simulink model "LTI_test"  (R2020b)
settings: Solver=VariableStepAuto  StartTime=0.0  StopTime=Tsim  RelTol=1e-3
values from neighbouring files (symbols this model uses):
  a = B(2,1)    [getMatrices.m]
  A = [0, 1, 0, 0 ... (first row only)    [ErrorStateMatrices.m]    (also in getMatrices.m = [)
  B = [Bswa Bcurv]    [ErrorStateMatrices.m]    (also in getMatrices.m = [0, 2*Cf/m, 0, 2*Cf*lf/Jz; 0, 0 , 0, 2*d*Csf/Jz]')
  Cf = VEHICLE.CORNERING_STIFF    [ErrorStateMatrices.m]    (also in LoadVehicleParameters.m = 72705; RunSimulation.m; getMatrices.m = 72705)
  collecting_data = controller_input(end)    [LTI_MPC.m]    (also in RunSimulation.m = 0)
  Cr = Cf    [ErrorStateMatrices.m]    (also in LoadVehicleParameters.m = 72705; RunSimulation.m; getMatrices.m = 72705)
  DLCoffset = round(vx*3.6/60*250,-1)    [RunSimulation.m]
  Iz = VEHICLE.INERTIA_Z    [RunSimulation.m]
  L = controller_input(end-2)    [LTI_MPC.m]    (also in RunSimulation.m = 15)
  lambda_alpha = 0.2    [RunSimulation.m]
  lambda_slack = 1e6    (= 1000000)    [RunSimulation.m]
  lf = VEHICLE.LF    [ErrorStateMatrices.m]    (also in LoadVehicleParameters.m = 1.311; RunSimulation.m; getMatrices.m = 1.311)
  lr = VEHICLE.LR    [ErrorStateMatrices.m]    (also in LoadVehicleParameters.m = 1.311; RunSimulation.m; getMatrices.m = 1.311)
  m = VEHICLE.MASS    [ErrorStateMatrices.m]    (also in LoadVehicleParameters.m = 1599.98; RunSimulation.m; getMatrices.m = 1599.98)
  N = T_test/Ts    (= 100)    [RunSimulation.m]    (also in nominalMPC.m = u(end))
  n = controller_input(end-1)    [LTI_MPC.m]    (also in RunSimulation.m = 4)
  nu = 2    [LTI_MPC.m]    (also in RunSimulation.m; nominalMPC.m = 1)
  ny = 2    [LTI_MPC.m]    (also in RunSimulation.m)
  Ts = 0.05    [RunSimulation.m]    (also in getMatrices.m = 0.1)
  vx = controller_input(2)    [LTI_MPC.m]    (also in RunSimulation.m = 22.2222222222)
undefined symbols (not defined in the file or in its folder): DDPC, DiscIntNeverNeededParam, nominalMPC, VEHICLE
libraries: simulink x2
settings Model: Creator=LAMES Workstation  LastModifiedBy=LAMES Workstation

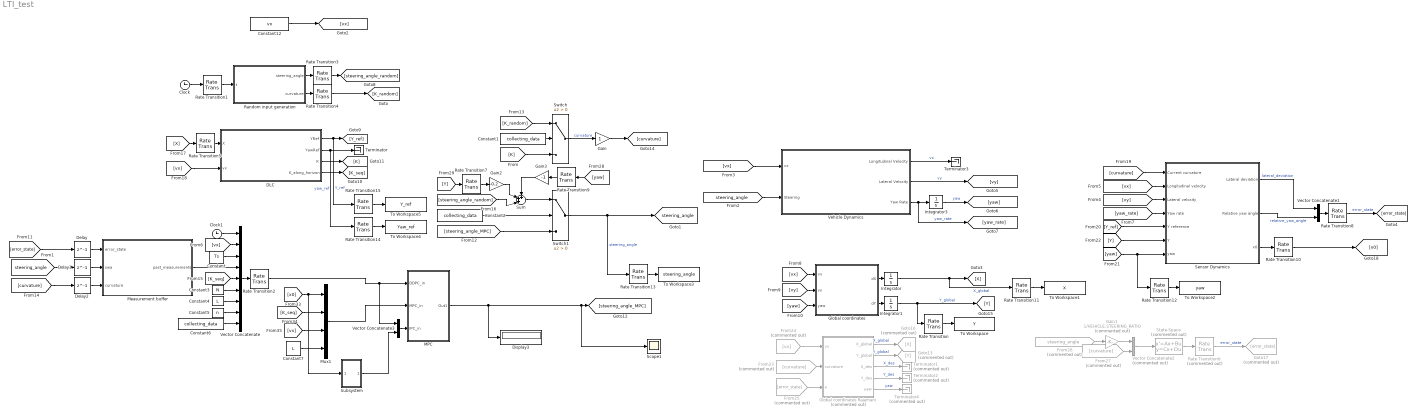
== system LTI_test ==
  Clock : Clock
  Clock1 : Clock
  Constant : Constant  Value=Ts  SampleTime=Ts
  Constant1 : Constant  Value=collecting_data  SampleTime=Ts
  Constant12 : Constant  Value=vx  SampleTime=Ts
  Constant2 : Constant  Value=collecting_data  SampleTime=Ts
  Constant3 : Constant  Value=N  SampleTime=Ts
  Constant4 : Constant  Value=L  SampleTime=Ts
  Constant5 : Constant  Value=n  SampleTime=Ts
  Constant6 : Constant  Value=collecting_data  SampleTime=Ts
  Constant7 : Constant  Value=L  SampleTime=Ts
  DLC : MATLAB Function  TreatAsAtomicUnit=on
  Delay : Delay  DelayLength=1  InitialCondition=0  SampleTime=Ts
  Delay1 : Delay  DelayLength=1  InitialCondition=0  SampleTime=Ts
  Delay2 : Delay  DelayLength=1  InitialCondition=0  SampleTime=Ts
  Display3 : Display
  From23 : From  Commented=on  GotoTag=curvature
  From24 : From  Commented=on  GotoTag=vx
  From25 : From  Commented=on  GotoTag=error_state
  From26 : From  Commented=on  GotoTag=steering_angle  TagVisibility=global
  From27 : From  Commented=on  GotoTag=curvature
  Gain : Gain
  Gain1 : Gain  Commented=on  Gain=1/VEHICLE.STEERING_RATIO
  Gain2 : Gain  Gain=-0.2
  Gain3 : Gain  Gain=-1
  Global coordinates : MATLAB Function  TreatAsAtomicUnit=on
  Global coordinates Rajamani : Subsystem  Commented=on
  Goto13 : Goto  Commented=on  GotoTag=Y
  Goto16 : Goto  Commented=on  GotoTag=X
  Goto17 : Goto  Commented=on  GotoTag=error_state
  Integrator : Integrator
  Integrator1 : Integrator
  Integrator3 : Integrator
  MPC : Subsystem  Variant=on
  Measurement buffer : MATLAB Function  TreatAsAtomicUnit=on
  Mux1 : Mux
  Random input generation : MATLAB Function  TreatAsAtomicUnit=on
  Rate Transition{,11..15} (6 alike) : RateTransition  InitialCondition=Ts
  Rate Transition1 : RateTransition  OutPortSampleTime="5*Ts  % hold the input for a few samples"
  Rate Transition{2..5,7..10} (8 alike) : RateTransition  OutPortSampleTime=Ts
  Rate Transition6 : RateTransition  Commented=on  OutPortSampleTime=Ts
  Scope1 : Scope
  Sensor Dynamics : Subsystem
  State-Space : StateSpace  Commented=on  A=A  B=B  C=[1 0 0 0; 0 0 1 0]  D=zeros(2)  InitialCondition=0
  Subsystem : Subsystem
  Sum : Sum  Inputs=+++|
  Switch : Switch  Criteria=u2 > Threshold
  Switch1 : Switch  Criteria=u2 > Threshold
  Terminator : Terminator
  Terminator1 : Terminator  Commented=on
  Terminator2 : Terminator  Commented=on
  Terminator3 : Terminator
  Terminator4 : Terminator  Commented=on
  To Workspace : ToWorkspace  VariableName=Y  SaveFormat=Timeseries  SampleTime=-1
  To Workspace1 : ToWorkspace  VariableName=X  SaveFormat=Timeseries  SampleTime=-1
  To Workspace2 : ToWorkspace  VariableName=yaw  SaveFormat=Timeseries  SampleTime=-1
  To Workspace3 : ToWorkspace  VariableName=steering_angle  SaveFormat=Timeseries  SampleTime=-1
  To Workspace4 : ToWorkspace  VariableName=Yaw_ref  SaveFormat=Timeseries  SampleTime=-1
  To Workspace5 : ToWorkspace  VariableName=Y_ref  SaveFormat=Timeseries  SampleTime=-1
  Vector Concatenate : Concatenate  NumInputs=9
  Vector Concatenate1 : Concatenate
  Vector Concatenate2 : Concatenate  Commented=on
  Vector Concatenate3 : Concatenate
  Vehicle Dynamics : Subsystem
  tag scope: steering_angle=global
  wires:
  Constant4/1 -> Vector Concatenate/7
  Constant5/1 -> Vector Concatenate/8
  [K_seq] -> Vector Concatenate/5
  Constant6/1 -> Vector Concatenate/9
  Constant3/1 -> Vector Concatenate/6
  Vector Concatenate/1 -> Rate Transition2/1
  [vx] -> Vector Concatenate/2
  Constant/1 -> Vector Concatenate/3
  Clock1/1 -> Vector Concatenate/1
  Measurement buffer/1(past_measurements) -> Vector Concatenate/4
  Constant1/1 -> Switch/2
  Gain/1 -> [curvature]
  [K_random] -> Switch/1
  [K] -> Switch/3
  Switch/1 -> Gain/1  "curvature"
  [steering_angle_MPC] -> Switch1/3
  Constant2/1 -> Switch1/2
  Switch1/1 -> Rate Transition13/1, [steering_angle]  "steering_angle"
  [steering_angle] -> Vehicle Dynamics/2(Steering)
  Vehicle Dynamics/1(Longitudinal Velocity) -> Terminator3/1  "vx"
  [vx] -> Vehicle Dynamics/1(vx)
  Constant12/1 -> [vx]
  [vy] -> Sensor Dynamics/3(Lateral velocity)
  [vx] -> Sensor Dynamics/2(Longitudinal velocity)
  [yaw_rate] -> Sensor Dynamics/4(Yaw rate)
  [yaw] -> Global coordinates/3(yaw)
  Integrator1/1 -> Rate Transition/1, [Y]  "Y_global"
  Global coordinates/2(dY) -> Integrator1/1
  Integrator/1 -> Rate Transition11/1, [X]  "X_global"
  [vx] -> Global coordinates/1(vx)
  [vy] -> Global coordinates/2(vy)
  Global coordinates/1(dX) -> Integrator/1
  Vector Concatenate1/1 -> Rate Transition8/1
  Sensor Dynamics/1(Lateral deviation) -> Vector Concatenate1/1  "lateral_deviation"
  Sensor Dynamics/2(Relative yaw angle) -> Vector Concatenate1/2  "relative_yaw_angle"
  DLC/3(K) -> [K]
  DLC/2(YawRef) -> Rate Transition14/1, Terminator/1  "yaw_ref"
  [vx] -> DLC/2(vx)
  DLC/4(K_along_horizon) -> [K_seq]
  DLC/1(YRef) -> Rate Transition15/1, [Y_ref]  "Y_ref"
  [curvature] -> Sensor Dynamics/1(Current curvature)
  Vehicle Dynamics/2(Lateral Velocity) -> [vy]  "vy"
  Integrator3/1 -> [yaw]  "yaw"
  Vehicle Dynamics/3(Yaw Rate) -> [yaw_rate], Integrator3/1  "yaw_rate"
  Rate Transition8/1 -> [error_state]  "error_state"
  [Y_ref] -> Sensor Dynamics/5(Y reference)
  [Y] -> Sensor Dynamics/6(Y)
  [yaw] -> Rate Transition12/1, Sensor Dynamics/7(yaw)
  [X] -> Rate Transition5/1
  Rate Transition5/1 -> DLC/1(X)
  From23/1 -> Global coordinates Rajamani/2(curvature)
  From24/1 -> Global coordinates Rajamani/1(vx)
  Global coordinates Rajamani/1(X_global) -> Goto16/1  "X_global"
  Global coordinates Rajamani/2(Y_global) -> Goto13/1  "Y_global"
  From25/1 -> Global coordinates Rajamani/3(e)
  Global coordinates Rajamani/3(X_des) -> Terminator1/1  "X_des"
  Global coordinates Rajamani/4(Y_des) -> Terminator2/1  "Y_des"
  From27/1 -> Vector Concatenate2/2
  Vector Concatenate2/1 -> State-Space/1
  State-Space/1 -> Rate Transition6/1
  Rate Transition6/1 -> Goto17/1  "error_state"
  Global coordinates Rajamani/5(yaw) -> Terminator4/1  "yaw"
  From26/1 -> Gain1/1
  Gain1/1 -> Vector Concatenate2/1
  Rate Transition2/1 -> Vector Concatenate3/1, MPC/1(DDPC_in)
  [error_state] -> Delay/1
  Delay/1 -> Measurement buffer/1(error_state)
  [steering_angle] -> Delay1/1
  Delay1/1 -> Measurement buffer/2(swa)
  [curvature] -> Delay2/1
  Delay2/1 -> Measurement buffer/3(curvature)
  [steering_angle_random] -> Sum/3
  Sum/1 -> Switch1/1
  Rate Transition7/1 -> Gain2/1
  Gain2/1 -> Sum/2
  [Y] -> Rate Transition7/1
  [yaw] -> Rate Transition9/1
  Rate Transition9/1 -> Gain3/1
  Gain3/1 -> Sum/1
  Sensor Dynamics/3(x0) -> Rate Transition10/1
  Rate Transition10/1 -> [x0]
  Rate Transition/1 -> To Workspace/1
  Rate Transition11/1 -> To Workspace1/1
  Rate Transition12/1 -> To Workspace2/1
  Rate Transition13/1 -> To Workspace3/1
  Rate Transition14/1 -> To Workspace4/1
  Rate Transition15/1 -> To Workspace5/1
  MPC/1(Out1) -> Display3/1, Scope1/1, [steering_angle_MPC]
  [vx] -> Mux1/3
  Mux1/1 -> MPC/2(MPC_in)
  [K_seq] -> Mux1/2
  [x0] -> Subsystem/1(In1), Mux1/1
  Rate Transition4/1 -> [K_random]
  Random input generation/2(curvature) -> Rate Transition4/1
  Clock/1 -> Rate Transition1/1
  Rate Transition3/1 -> [steering_angle_random]
  Rate Transition1/1 -> Random input generation/1(t)
  Random input generation/1(steering_angle) -> Rate Transition3/1
  Constant7/1 -> Mux1/4
  Vector Concatenate3/1 -> MPC/3(IPC_in)
  Subsystem/1(Out1) -> Vector Concatenate3/2

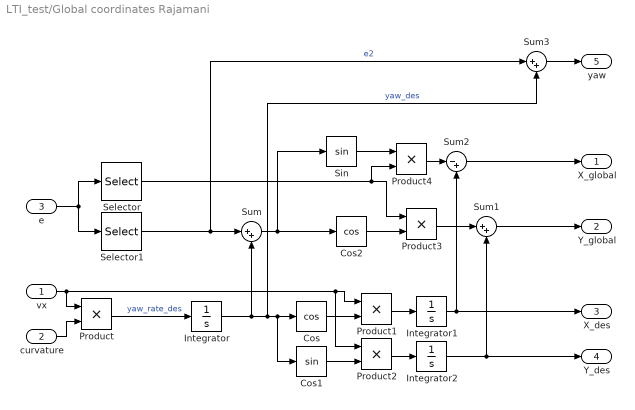
== system LTI_test/Global coordinates Rajamani ==
  vx : Inport
  curvature : Inport  Port=2
  e : Inport  Port=3
  Cos : Trigonometry  Operator=cos
  Cos1 : Trigonometry
  Cos2 : Trigonometry  Operator=cos
  Integrator : Integrator
  Integrator1 : Integrator
  Integrator2 : Integrator
  Product{,1..4} (5 alike) : Product
  Selector : Selector  InputPortWidth=2  IndexOptions=Index vector (dialog)  Indices=1  OutputSizes=1
  Selector1 : Selector  InputPortWidth=2  IndexOptions=Index vector (dialog)  Indices=2  OutputSizes=1
  Sin : Trigonometry
  Sum : Sum  Inputs=|++
  Sum1 : Sum  Inputs=|++
  Sum2 : Sum  Inputs=|-+
  Sum3 : Sum  Inputs=|++
  X_global : Outport
  Y_global : Outport  Port=2
  X_des : Outport  Port=3
  Y_des : Outport  Port=4
  yaw : Outport  Port=5
  wires:
  vx/1 -> Product2/1, Product1/1, Product/1
  curvature/1 -> Product/2
  Product/1 -> Integrator/1  "yaw_rate_des"
  Integrator/1 -> Sum/2, Sum3/2, Cos1/1, Cos/1  "yaw_des"
  Cos/1 -> Product1/2
  Cos1/1 -> Product2/2
  Product2/1 -> Integrator2/1
  Product1/1 -> Integrator1/1
  e/1 -> Selector1/1, Selector/1
  Selector1/1 -> Sum3/1, Sum/1  "e2"
  Sum/1 -> Sin/1, Cos2/1
  Cos2/1 -> Product3/2
  Selector/1 -> Product4/2, Product3/1
  Product3/1 -> Sum1/1
  Product4/1 -> Sum2/1
  Sin/1 -> Product4/1
  Sum2/1 -> X_global/1
  Sum1/1 -> Y_global/1
  Integrator1/1 -> X_des/1, Sum2/2
  Integrator2/1 -> Y_des/1, Sum1/2
  Sum3/1 -> yaw/1

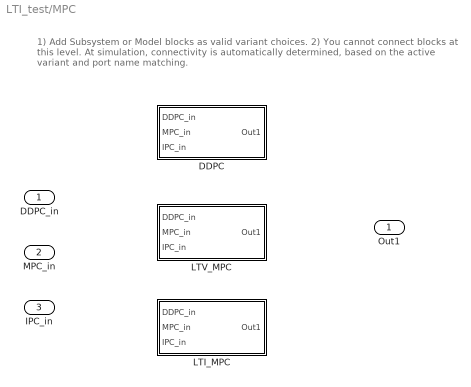
== system LTI_test/MPC ==
  note: 1) Add Subsystem or Model blocks as valid variant choices.
      | 2) You cannot connect blocks at this level. At simulation, connectivity is automatically
      | determined, based on the active variant and port name matching.
  DDPC_in : Inport
  MPC_in : Inport  Port=2
  IPC_in : Inport  Port=3
  DDPC : Subsystem  VariantControl=mpc_variant == 0
  LTI_MPC : Subsystem  VariantControl=mpc_variant == 2
  LTV_MPC : Subsystem  VariantControl=mpc_variant == 1
  Out1 : Outport

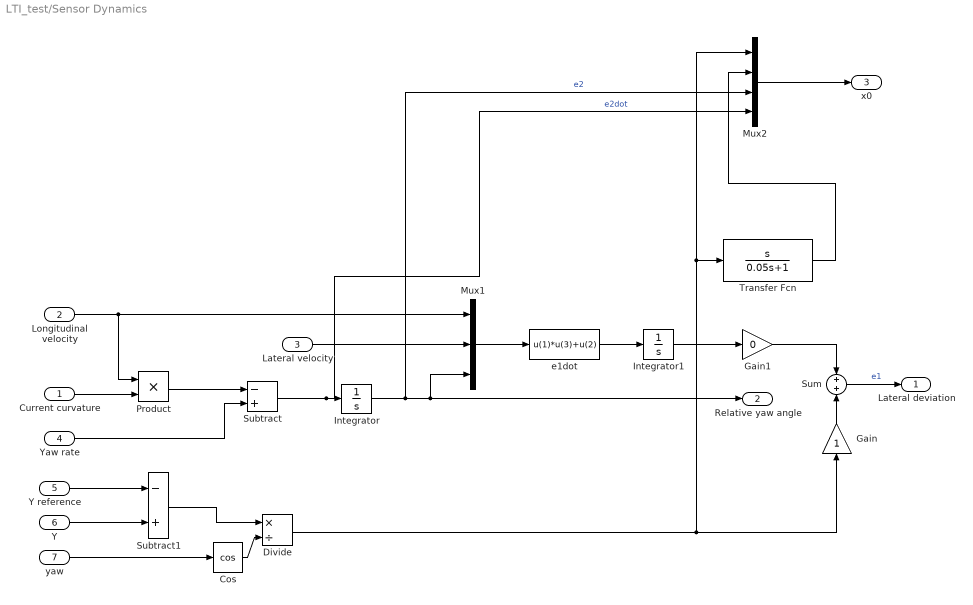
== system LTI_test/Sensor Dynamics ==
  Current curvature : Inport
  Longitudinal velocity : Inport  Port=2
  Lateral velocity : Inport  Port=3
  Yaw rate : Inport  Port=4
  Y reference : Inport  Port=5
  Y : Inport  Port=6
  yaw : Inport  Port=7
  Cos : Trigonometry  Operator=cos
  Divide : Product  Inputs=*/
  Gain : Gain
  Gain1 : Gain  Gain=0
  Integrator : Integrator
  Integrator1 : Integrator
  Mux1 : Mux  Inputs=[1 1 1]
  Mux2 : Mux
  Product : Product
  Subtract : Sum  Inputs=-+
  Subtract1 : Sum  Inputs=-+
  Sum : Sum  Inputs=+|+
  Transfer Fcn : TransferFcn  Numerator=[1 0]  Denominator=[0.05 1]
  e1dot : Fcn  Expr=u(1)*u(3)+u(2)
  Lateral deviation : Outport  VectorParamsAs1DForOutWhenUnconnected=off
  Relative yaw angle : Outport  Port=2  VectorParamsAs1DForOutWhenUnconnected=off
  x0 : Outport  Port=3  VectorParamsAs1DForOutWhenUnconnected=off
  wires:
  Current curvature/1 -> Product/2
  Mux1/1 -> e1dot/1
  Longitudinal velocity/1 -> Product/1, Mux1/1
  Lateral velocity/1 -> Mux1/2
  Product/1 -> Subtract/1
  Yaw rate/1 -> Subtract/2
  Y/1 -> Subtract1/2
  Subtract1/1 -> Divide/1
  yaw/1 -> Cos/1
  Cos/1 -> Divide/2
  Y reference/1 -> Subtract1/1
  Integrator1/1 -> Gain1/1
  Gain/1 -> Sum/2
  Gain1/1 -> Sum/1
  Sum/1 -> Lateral deviation/1  "e1"
  e1dot/1 -> Integrator1/1
  Mux2/1 -> x0/1
  Integrator/1 -> Mux2/3, Mux1/3, Relative yaw angle/1  "e2"
  Subtract/1 -> Mux2/4, Integrator/1  "e2dot"
  Divide/1 -> Mux2/1, Transfer Fcn/1, Gain/1
  Transfer Fcn/1 -> Mux2/2

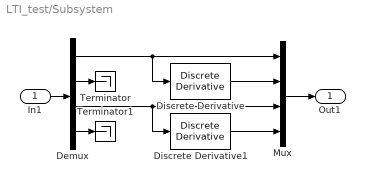
== system LTI_test/Subsystem ==
  In1 : Inport
  Demux : Demux
  Discrete Derivative : simulink/Quick Insert/Discrete/Discrete Derivative  gainval=1.0  ICPrevScaledInput=0.0  OutMin=[]  OutMax=[]  OutDataType=fixdt(1, 16)  OutScaling=2^-10  DoSatur=off
      settings: SourceProductBaseCode=SL
  Discrete Derivative1 : simulink/Quick Insert/Discrete/Discrete Derivative  gainval=1.0  ICPrevScaledInput=0.0  OutMin=[]  OutMax=[]  OutDataType=fixdt(1, 16)  OutScaling=2^-10  DoSatur=off
      settings: SourceProductBaseCode=SL
  Mux : Mux
  Terminator : Terminator
  Terminator1 : Terminator
  Out1 : Outport
  wires:
  Demux/4 -> Terminator1/1
  Demux/1 -> Discrete Derivative/1, Mux/1
  Discrete Derivative1/1 -> Mux/4
  Demux/3 -> Discrete Derivative1/1, Mux/3
  Discrete Derivative/1 -> Mux/2
  Mux/1 -> Out1/1
  In1/1 -> Demux/1
  Demux/2 -> Terminator/1

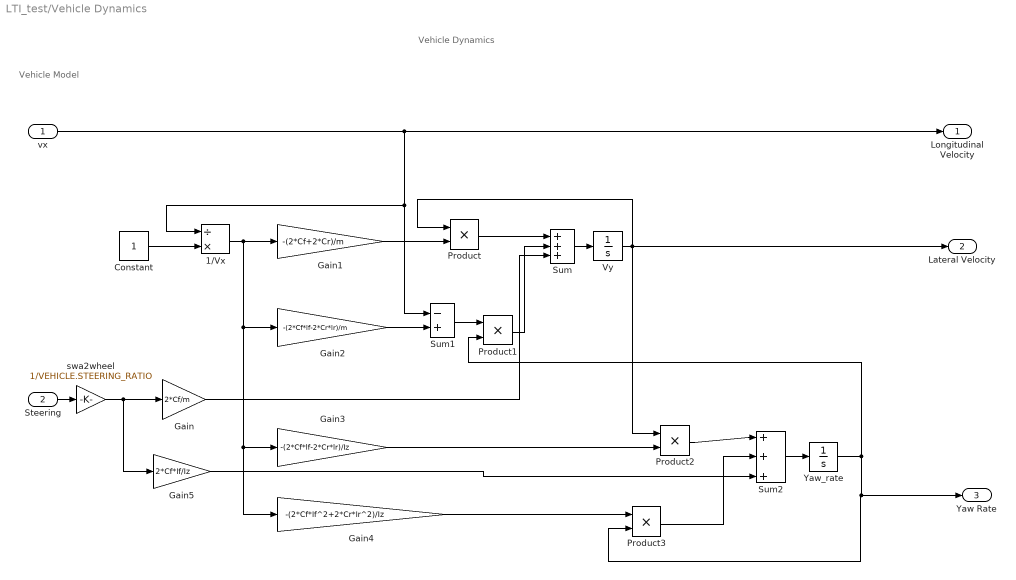
== system LTI_test/Vehicle Dynamics ==
  note: Vehicle Model
  note: Vehicle Dynamics
  vx : Inport
  Steering : Inport  Port=2
  1/Vx : Product  Inputs=/*
  Constant : Constant
  Gain : Gain  Gain=2*Cf/m
  Gain1 : Gain  Gain=-(2*Cf+2*Cr)/m
  Gain2 : Gain  Gain=-(2*Cf*lf-2*Cr*lr)/m
  Gain3 : Gain  Gain=-(2*Cf*lf-2*Cr*lr)/Iz
  Gain4 : Gain  Gain=-(2*Cf*lf^2+2*Cr*lr^2)/Iz
  Gain5 : Gain  Gain=2*Cf*lf/Iz
  Product{,1..3} (4 alike) : Product
  Sum : Sum  Inputs=+++
  Sum1 : Sum  Inputs=-+
  Sum2 : Sum  Inputs=+++
  Vy : Integrator
  "Yaw_rate " : Integrator
  swa2wheel : Gain  Gain=1/VEHICLE.STEERING_RATIO
  Longitudinal Velocity : Outport  VectorParamsAs1DForOutWhenUnconnected=off
  Lateral Velocity : Outport  Port=2  VectorParamsAs1DForOutWhenUnconnected=off
  Yaw Rate : Outport  Port=3  VectorParamsAs1DForOutWhenUnconnected=off
  wires:
  Sum2/1 -> "Yaw_rate "/1
  Gain2/1 -> Sum1/2
  Gain4/1 -> Product3/1
  Constant/1 -> 1/Vx/2
  Gain3/1 -> Product2/2
  1/Vx/1 -> Gain4/1, Gain3/1, Gain2/1, Gain1/1
  Product2/1 -> Sum2/1
  Product3/1 -> Sum2/2
  Gain5/1 -> Sum2/3
  Sum1/1 -> Product1/1
  "Yaw_rate "/1 -> Yaw Rate/1, Product3/2, Product1/2
  Gain/1 -> Sum/3
  Steering/1 -> swa2wheel/1
  Gain1/1 -> Product/2
  Product/1 -> Sum/1
  Vy/1 -> Product/1, Lateral Velocity/1, Product2/1
  Sum/1 -> Vy/1
  vx/1 -> 1/Vx/1, Sum1/1, Longitudinal Velocity/1
  Product1/1 -> Sum/2
  swa2wheel/1 -> Gain/1, Gain5/1

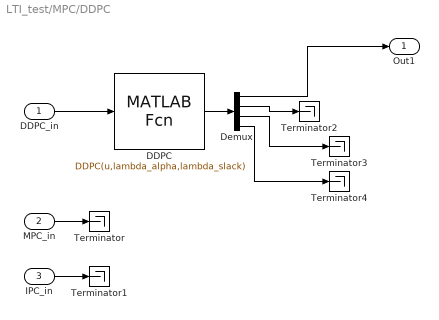
== system LTI_test/MPC/DDPC ==
  DDPC_in : Inport
  MPC_in : Inport  Port=2
  IPC_in : Inport  Port=3
  DDPC : MATLABFcn  MATLABFcn=DDPC(u,lambda_alpha,lambda_slack)  OutputDimensions=4
  Demux : Demux
  Terminator{,1..4} (5 alike) : Terminator
  Out1 : Outport
  wires:
  MPC_in/1 -> Terminator/1
  DDPC_in/1 -> DDPC/1
  Demux/1 -> Out1/1
  DDPC/1 -> Demux/1
  Demux/2 -> Terminator2/1
  Demux/3 -> Terminator3/1
  Demux/4 -> Terminator4/1
  IPC_in/1 -> Terminator1/1

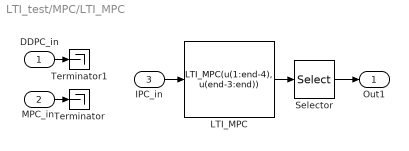
== system LTI_test/MPC/LTI_MPC ==
  DDPC_in : Inport
  MPC_in : Inport  Port=2
  IPC_in : Inport  Port=3
  LTI_MPC : MATLABFcn  MATLABFcn=LTI_MPC(u(1:end-4), u(end-3:end))  OutputDimensions=4
  Selector : Selector  InputPortWidth=4  IndexOptions=Index vector (dialog)  Indices=1  OutputSizes=1
  Terminator : Terminator
  Terminator1 : Terminator
  Out1 : Outport
  wires:
  LTI_MPC/1 -> Selector/1
  MPC_in/1 -> Terminator/1
  IPC_in/1 -> LTI_MPC/1
  DDPC_in/1 -> Terminator1/1
  Selector/1 -> Out1/1

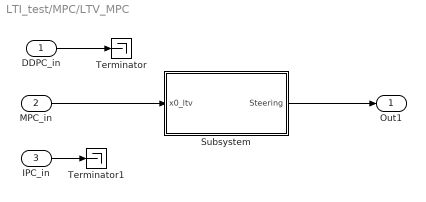
== system LTI_test/MPC/LTV_MPC ==
  DDPC_in : Inport
  MPC_in : Inport  Port=2
  IPC_in : Inport  Port=3
  Subsystem : Subsystem
  Terminator : Terminator
  Terminator1 : Terminator
  Out1 : Outport
  wires:
  Subsystem/1(Steering) -> Out1/1
  DDPC_in/1 -> Terminator/1
  MPC_in/1 -> Subsystem/1(x0_ltv)
  IPC_in/1 -> Terminator1/1

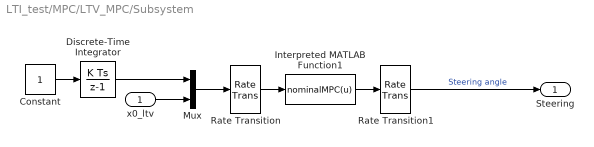
== system LTI_test/MPC/LTV_MPC/Subsystem ==
  x0_ltv : Inport
  Constant : Constant
  Discrete-Time Integrator : DiscreteIntegrator  SampleTime=-1  ICPrevOutput=DiscIntNeverNeededParam  ICPrevScaledInput=DiscIntNeverNeededParam
  Interpreted MATLAB Function1 : MATLABFcn  MATLABFcn=nominalMPC(u)  OutputDimensions=1
  Mux : Mux  Inputs=2
  Rate Transition : RateTransition  OutPortSampleTime=Ts
  Rate Transition1 : RateTransition  OutPortSampleTime=Ts
  Steering : Outport
  wires:
  Interpreted MATLAB Function1/1 -> Rate Transition1/1
  Rate Transition/1 -> Interpreted MATLAB Function1/1
  Rate Transition1/1 -> Steering/1  "Steering angle"
  x0_ltv/1 -> Mux/2
  Mux/1 -> Rate Transition/1
  Discrete-Time Integrator/1 -> Mux/1
  Constant/1 -> Discrete-Time Integrator/1

== matlab function LTI_test/Measurement buffer ==
  data: error_state input; swa input; curvature input; past_measurements output; n parameter; ny parameter; nu parameter
function past_measurements = remember(error_state,swa,curvature,n,ny,nu)
% a function for saving n past input/output measurements
persistent yupast
if (isempty(yupast))
    yupast = zeros(ny+nu, n);
end
yupast = circshift(yupast,-1,2);  % shift columns left by one step
yupast(:,end) = [error_state;swa;curvature];  % add last measurements to the end
past_measurements = yupast(:);  % unroll
end

== matlab function LTI_test/Random input generation ==
  data: t input; steering_angle output; curvature output
function [steering_angle, curvature] = RandomInput(t)
swa_min = -90; swa_max = 90;  % degrees
swa_min = deg2rad(swa_min); swa_max = deg2rad(swa_max);
curvature_min = -0.02; curvature_max = 0.02;  % from the DLC maneuver
if (t>15 && t<30)
    steering_angle = swa_min + (swa_max-swa_min)*rand(1);
    curvature = curvature_min + (curvature_max-curvature_min)*rand(1);
else
    steering_angle = 0;
    curvature = 0;
end

== matlab function LTI_test/DLC ==
  data: X input; YRef output; YawRef output; K output; K_along_horizon output; vx input; L parameter; DLCoffset parameter; Ts parameter
function [YRef, YawRef, K, K_along_horizon] = DoubleLaneChange(X, vx, L, DLCoffset, Ts)
% https://de.mathworks.com/help/mpc/ug/lane-keeping-assist-system-using-model-predictive-control.html
% https://www.semanticscholar.org/paper/MPC-Based-Approach-to-Active-Steering-for-Vehicle-Borrelli-Falcone/0b96422c76cd7e1ae584d25de26a41a7b1505a40
% L is the prediction horizon
% DLCoffset defines the X at which the maneuver starts

X_along_horizon = linspace(X, X+vx*L*Ts, L+2);

shape = 2.4;
dx1 = 25;
dx2 = 21.95;
dy1 = 4.05;
dy2 = 5.7;
Xs1 = 27.19;
Xs2 = 56.45;

z1 = shape/dx1*(X_along_horizon - DLCoffset - Xs1) - shape/2;
z2 = shape/dx2*(X_along_horizon - DLCoffset - Xs2) - shape/2;

yaw_along_horizon = atan( dy1*(1./cosh(z1)).^2*(1.2/dx1) - dy2*(1./cosh(z2)).^2*(1.2/dx2));
Y_along_horizon = dy1/2*(1+tanh(z1)) - dy2/2*(1+tanh(z2));

YawRef = yaw_along_horizon(1);
YRef = Y_along_horizon(1);

% Petrova formula
% K = -((dy1*shape^2*tanh(shape/2 - (shape*(X - DLCoffset - Xs1))/dx1)*(tanh(shape/2 - (shape*(X - DLCoffset - Xs1))/dx1)^2 - 1))/dx1^2 - (dy2*shape^2*tanh(shape/2 - (shape*(X - DLCoffset - Xs2))/dx2)*(tanh(shape/2 - (shape*(X - DLCoffset - Xs2))/dx2)^2 - 1))/dx2^2)/(((dy1*shape*(tanh(shape/2 - (shape*(X - DLCoffset - Xs1))/dx1)^2 - 1))/(2*dx1) - (dy2*shape*(tanh(shape/2 - (shape*(X - DLCoffset - Xs2))/dx2)^2 - 1))/(2*dx2))^2 + 1)^(3/2);
% K_along_horizon = -((dy1.*shape.^2.*tanh(shape./2 - (shape.*(X_along_horizon - DLCoffset - Xs1))./dx1).*(tanh(shape./2 - (shape.*(X_along_horizon - DLCoffset - Xs1))./dx1).^2 - 1))./dx1.^2 - (dy2.*shape.^2.*tanh(shape./2 - (shape.*(X_along_horizon - DLCoffset - Xs2))./dx2).*(tanh(shape./2 - (shape.*(X_along_horizon - DLCoffset - Xs2))./dx2).^2 - 1))./dx2.^2)./(((dy1.*shape.*(tanh(shape./2 - (shape.*(X_along_horizon - DLCoffset - Xs1))./dx1).^2 - 1))./(2.*dx1) - (dy2.*shape.*(tanh(shape./2 - (shape.*(X_along_horizon - DLCoffset - Xs2))./dx2).^2 - 1))./(2.*dx2)).^2 + 1).^(3./2);

% Desired curvature (MPC toolbox, modified)
DX = diff(X_along_horizon) / Ts; 
% DX = [DX, DX(end)];
DY = diff(Y_along_horizon) / Ts;
D2Y = diff(DY) / Ts; 
DX = DX(1:L);
DY = DY(1:L);
D2Y = D2Y(1:L);
% DY = [DY, DY(end)];
% D2Y = [D2Y, D2Y(end), D2Y(end)];

if vx == 0
    K_along_horizon = zeros(size(DX));
    K = 0;
else
    K_along_horizon = DX.*D2Y./(DX.^2+DY.^2).^(3/2);
    K = K_along_horizon(1);
end

% K_along_horizon = K_along_horizon(1:L);
end

== matlab function LTI_test/Global coordinates ==
  data: vx input; dX output; vy input; yaw input; dY output
function [dX, dY] = GlobalCoordinates(vx,vy,yaw)
    
    dX = vx.*cos(yaw) - vy.*sin(yaw);
    dY = vx.*sin(yaw) + vy.*cos(yaw);

end
